simulink model "z8"  (R2023b)
settings: Solver=FixedStepAuto  StartTime=0.0  StopTime=10.0  FixedStep=0.01  RelTol=1e-3
values from neighbouring files (symbols this model uses):
  C = q_bar * S * C_C    [z8.m]
  D = q_bar * S * C_D    [z8.m]
  L = q_bar * S * C_L    [z8.m]
undefined symbols (not defined in the file or in its folder): Ix, Iy, Iz, l_AB, m_AB, n_AB
settings Model: Creator=asus  LastModifiedBy=asus

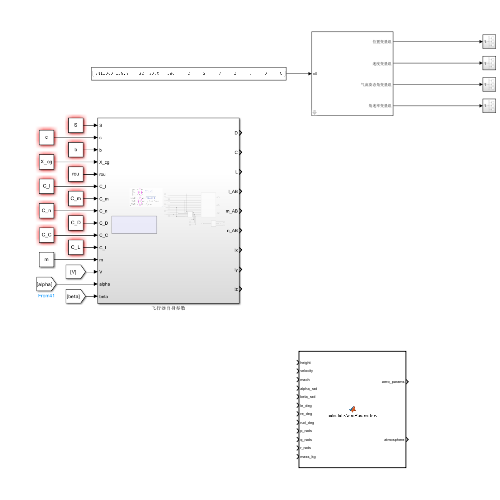
[thumbnail: Simulink's stored preview of the top-level diagram]
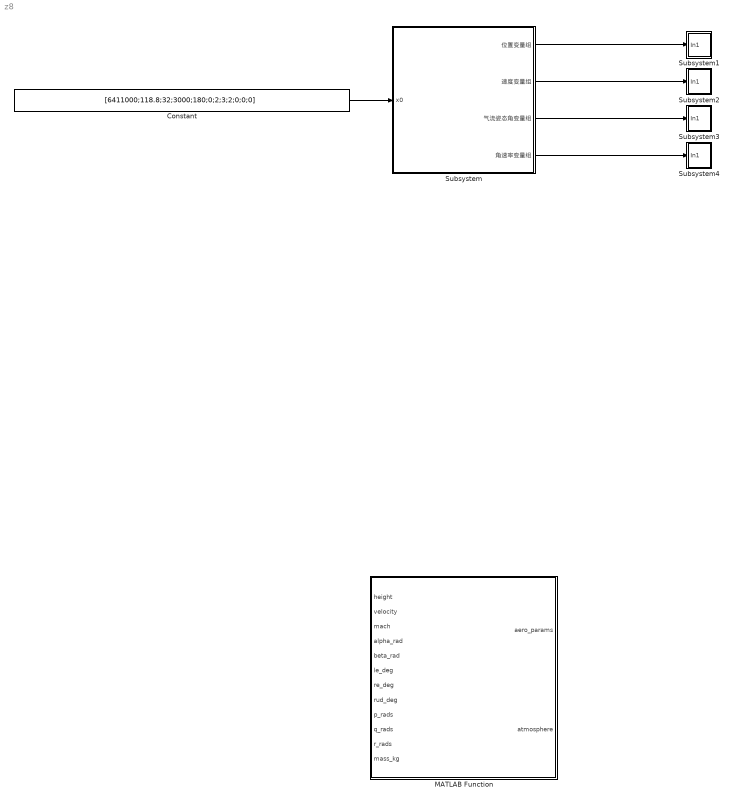
== system z8 ==
  Constant : Constant  Value=[6411000;118.8;32;3000;180;0;2;3;2;0;0;0]
  MATLAB Function : MATLAB Function  TreatAsAtomicUnit=on
  Subsystem : Subsystem  mask{m=136820, g=9.65, w_E=7.3*1e-5, S=334.73, c=24.384, b=18.288, rou=0, C_I=0, C_m=0, C_n=0, C_D=0, C_C=0, C_L=0}
      mask prompts: m "m质量"; g "g重力加速度"; w_E "w_E地球自转角速度"; S "S机翼面积"; c "c平均气动弦长"; b "b机翼展长"; C_I "C_l"
      mask DialogControl ParameterGroupVar Prompt: 参数
  Subsystem1 : Subsystem
  Subsystem2 : Subsystem
  Subsystem3 : Subsystem
  Subsystem4 : Subsystem
  wires:
  Constant/1 -> Subsystem/1(x0)
  Subsystem/2(速度变量组) -> Subsystem2/1(In1)
  Subsystem/4(角速率变量组) -> Subsystem4/1(In1)
  Subsystem/1(位置变量组) -> Subsystem1/1(In1)
  Subsystem/3(气流姿态角变量组) -> Subsystem3/1(In1)

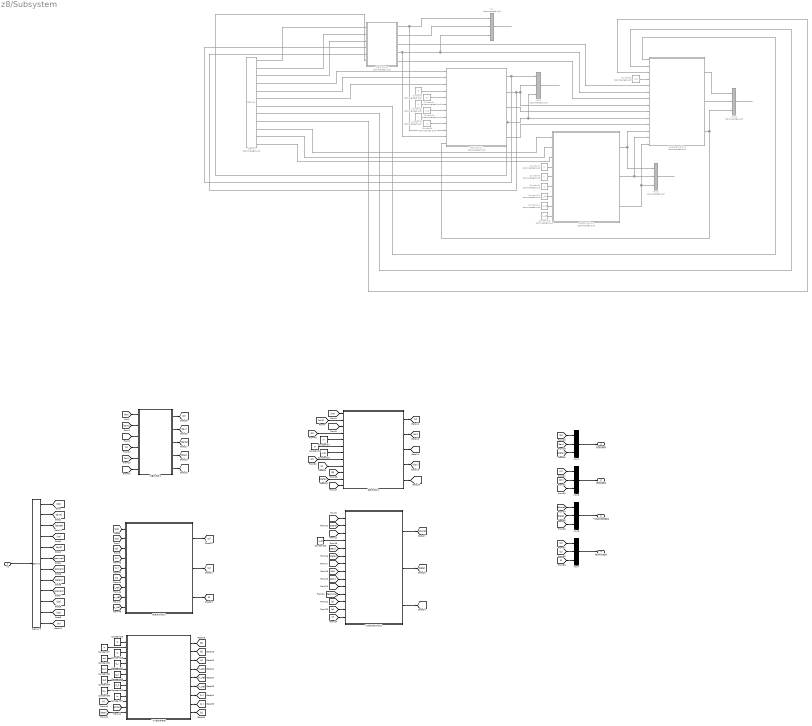
== system z8/Subsystem ==
  x0 : Inport
  Constant : Constant  Commented=on  Value=D
  Constant1 : Constant  Commented=on  Value=m
  Constant10 : Constant  Commented=on  Value=l_AB
  Constant11 : Constant  Commented=on  Value=m_AB
  Constant12 : Constant  Commented=on  Value=n_AB
  Constant14 : Constant  Value=m
  Constant18 : Constant  Value=g
  Constant19 : Constant  Value=w_E
  Constant2 : Constant  Commented=on  Value=g
  Constant22 : Constant  Value=w_E
  Constant26 : Constant  Value=S
  Constant27 : Constant  Value=c
  Constant28 : Constant  Value=b
  Constant3 : Constant  Commented=on  Value=w_E
  Constant30 : Constant  Value=rou
  Constant31 : Constant  Value=C_I
  Constant32 : Constant  Value=C_m
  Constant33 : Constant  Value=C_n
  Constant34 : Constant  Value=C_D
  Constant35 : Constant  Value=C_C
  Constant36 : Constant  Value=C_L
  Constant37 : Constant  Value=m
  Constant4 : Constant  Commented=on  Value=L
  Constant5 : Constant  Commented=on  Value=C
  Constant6 : Constant  Commented=on  Value=w_E
  Constant7 : Constant  Commented=on  Value=Ix
  Constant8 : Constant  Commented=on  Value=Iy
  Constant9 : Constant  Commented=on  Value=Iz
  Demux : Demux  Commented=on  Outputs=12
  Demux1 : Demux  Outputs=12
  Mux{,1..3} (4 alike) : Mux  Commented=on  Inputs=3
  Mux{4..7} (4 alike) : Mux  Inputs=3
  位置方程组1 : Subsystem
  位置方程组12 : Subsystem  Commented=on
  气流姿态角方程组1 : Subsystem
  气流姿态角方程组12 : Subsystem  Commented=on
  角速率方程组1 : Subsystem
  角速率方程组12 : Subsystem  Commented=on
  速度方程组1 : Subsystem
  速度方程组12 : Subsystem  Commented=on
  飞行器自身参数 : Subsystem
  位置变量组 : Outport
  速度变量组 : Outport  Port=2
  气流姿态角变量组 : Outport  Port=3
  角速率变量组 : Outport  Port=4
  wires:
  气流姿态角方程组12/2(beta) -> Mux2/2
  角速率方程组12/1(p) -> Mux3/1, 气流姿态角方程组12/12(p)
  Constant12/1 -> 角速率方程组12/9(n_AB)
  Demux/11 -> 角速率方程组12/2(q0)
  Constant2/1 -> 速度方程组12/6(g)
  位置方程组12/1(R) -> Mux/1, 速度方程组12/10(R)
  角速率方程组12/2(q) -> Mux3/2, 气流姿态角方程组12/13(q)
  Demux/5 -> 速度方程组12/2(chi0)
  Demux/1 -> 位置方程组12/1(R0)
  位置方程组12/4(delta) -> 气流姿态角方程组12/6(delta), Mux/3, 速度方程组12/11(delta)
  速度方程组12/1(V) -> 位置方程组12/4(V), Mux1/1
  Constant4/1 -> 速度方程组12/8(L)
  Mux2/1 -> ?
  角速率方程组12/3(r) -> Mux3/3, 气流姿态角方程组12/14(r)
  Constant8/1 -> 角速率方程组12/5(Iy)
  Demux/2 -> 位置方程组12/2(tau0)
  速度方程组12/2(chi) -> 位置方程组12/5(chi), Mux1/2, 气流姿态角方程组12/8(chi)
  气流姿态角方程组12/1(alpha) -> Mux2/1
  气流姿态角方程组12/3(sigma) -> Mux2/3, 速度方程组12/12(sigma)
  速度方程组12/4(gamma) -> 位置方程组12/6(gamma), Mux1/3, 气流姿态角方程组12/10(gamma)
  Mux3/1 -> ?
  位置方程组12/2(tau) -> Mux/2
  Constant7/1 -> 角速率方程组12/4(Ix)
  Demux/6 -> 速度方程组12/3(gamma0)
  Constant1/1 -> 速度方程组12/5(m)
  Demux/10 -> 角速率方程组12/1(p0)
  速度方程组12/5(dgamma) -> 气流姿态角方程组12/11(dgamma)
  Constant11/1 -> 角速率方程组12/8(m_AB)
  位置方程组12/3(dtau) -> 气流姿态角方程组12/5(dtau)
  Demux/4 -> 速度方程组12/1(V0)
  Mux1/1 -> ?
  Demux/12 -> 角速率方程组12/3(r0)
  位置方程组12/5(dddelta) -> 气流姿态角方程组12/7(ddelta)
  速度方程组12/3(dchi) -> 气流姿态角方程组12/9(dchi)
  Constant5/1 -> 速度方程组12/9(C)
  Constant6/1 -> 气流姿态角方程组12/4(w_E)
  Constant/1 -> 速度方程组12/4(D)
  Constant9/1 -> 角速率方程组12/6(Iz)
  Demux/8 -> 气流姿态角方程组12/2(beta0)
  Mux/1 -> ?
  Constant3/1 -> 速度方程组12/7(w_E)
  Constant10/1 -> 角速率方程组12/7(l_AB)
  Demux/9 -> 气流姿态角方程组12/3(sigma0)
  ? -> Demux/1
  Demux/3 -> 位置方程组12/3(delta0)
  Demux/7 -> 气流姿态角方程组12/1(alpha0)
  [C] -> 速度方程组1/8(L)
  Mux5/1 -> 速度变量组/1
  x0/1 -> Demux1/1
  Constant22/1 -> 气流姿态角方程组1/4(w_E)
  [Ix] -> 角速率方程组1/4(Ix)
  Mux7/1 -> 角速率变量组/1
  [L] -> 速度方程组1/9(C)
  Constant14/1 -> 速度方程组1/5(m)
  Constant19/1 -> 速度方程组1/7(w_E)
  Mux6/1 -> 气流姿态角变量组/1
  [D] -> 速度方程组1/4(D)
  Constant18/1 -> 速度方程组1/6(g)
  Demux1/1 -> [R0]
  Demux1/2 -> [tau0]
  Demux1/3 -> [delta0]
  Demux1/4 -> [V0]
  Demux1/5 -> [chi0]
  Demux1/6 -> [gamma0]
  Demux1/7 -> [alpha0]
  Demux1/8 -> [beta0]
  Demux1/9 -> [sigma0]
  Demux1/10 -> [p0]
  Demux1/11 -> [q0]
  Demux1/12 -> [r0]
  [R0] -> 位置方程组1/1(R0)
  [tau0] -> 位置方程组1/2(tau0)
  [delta0] -> 位置方程组1/3(delta0)
  [V0] -> 速度方程组1/1(V0)
  [chi0] -> 速度方程组1/2(chi0)
  [gamma0] -> 速度方程组1/3(gamma0)
  [p0] -> 角速率方程组1/1(p0)
  [q0] -> 角速率方程组1/2(q0)
  [r0] -> 角速率方程组1/3(r0)
  [alpha0] -> 气流姿态角方程组1/1(alpha0)
  [beta0] -> 气流姿态角方程组1/2(beta0)
  [sigma0] -> 气流姿态角方程组1/3(sigma0)
  速度方程组1/1(V) -> [V]
  速度方程组1/2(chi) -> [chi]
  速度方程组1/3(gamma) -> [gamma]
  [V] -> 位置方程组1/4(V)
  [chi] -> 位置方程组1/5(chi)
  [gamma] -> 位置方程组1/6(gamma)
  位置方程组1/4(dtau) -> [dtau]
  位置方程组1/5(dddelta) -> [ddelta]
  位置方程组1/3(delta) -> [delta]
  位置方程组1/1(R) -> [R]
  [dtau] -> 气流姿态角方程组1/5(dtau)
  [delta] -> 气流姿态角方程组1/6(delta)
  [ddelta] -> 气流姿态角方程组1/7(ddelta)
  [chi] -> 气流姿态角方程组1/8(chi)
  [dchi] -> 气流姿态角方程组1/9(dchi)
  速度方程组1/4(dchi) -> [dchi]
  速度方程组1/5(dgamma) -> [dgamma]
  [gamma] -> 气流姿态角方程组1/10(gamma)
  [dgamma] -> 气流姿态角方程组1/11(dgamma)
  角速率方程组1/1(p) -> [p]
  角速率方程组1/2(q) -> [q]
  角速率方程组1/3(r) -> [r]
  [p] -> 气流姿态角方程组1/12(p)
  [q] -> 气流姿态角方程组1/13(q)
  [r] -> 气流姿态角方程组1/14(r)
  [R] -> 速度方程组1/10(R)
  [delta] -> 速度方程组1/11(delta)
  [sigma] -> 速度方程组1/12(sigma)
  气流姿态角方程组1/3(sigma) -> [sigma]
  位置方程组1/2(tau) -> [tau]
  气流姿态角方程组1/2(beta) -> [beta]
  气流姿态角方程组1/1(alpha) -> [alpha]
  Mux4/1 -> 位置变量组/1
  [R] -> Mux4/1
  [tau] -> Mux4/2
  [delta] -> Mux4/3
  [V] -> Mux5/1
  [chi] -> Mux5/2
  [gamma] -> Mux5/3
  [alpha] -> Mux6/1
  [beta] -> Mux6/2
  [sigma] -> Mux6/3
  [p] -> Mux7/1
  [q] -> Mux7/2
  [r] -> Mux7/3
  Constant26/1 -> 飞行器自身参数/1(S)
  Constant27/1 -> 飞行器自身参数/2(c)
  Constant28/1 -> 飞行器自身参数/3(b)
  Constant30/1 -> 飞行器自身参数/4(rou)
  Constant31/1 -> 飞行器自身参数/5(C_l)
  Constant32/1 -> 飞行器自身参数/6(C_m)
  Constant33/1 -> 飞行器自身参数/7(C_n)
  Constant34/1 -> 飞行器自身参数/8(C_D)
  Constant35/1 -> 飞行器自身参数/9(C_C)
  Constant36/1 -> 飞行器自身参数/10(C_L)
  Constant37/1 -> 飞行器自身参数/11(m)
  [V] -> 飞行器自身参数/12(V)
  [alpha] -> 飞行器自身参数/13(alpha)
  [beta] -> 飞行器自身参数/14(beta)
  飞行器自身参数/1(D) -> [D]
  飞行器自身参数/2(C) -> [C]
  飞行器自身参数/3(L) -> [L]
  飞行器自身参数/4(l_AB) -> [l_AB]
  飞行器自身参数/5(m_AB) -> [m_AB]
  飞行器自身参数/6(n_AB) -> [n_AB]
  飞行器自身参数/7(Ix) -> [Ix]
  飞行器自身参数/8(Iy) -> [Iy]
  飞行器自身参数/9(Iz) -> [Iz]
  [Iy] -> 角速率方程组1/5(Iy)
  [Iz] -> 角速率方程组1/6(Iz)
  [l_AB] -> 角速率方程组1/7(l_AB)
  [m_AB] -> 角速率方程组1/8(m_AB)
  [n_AB] -> 角速率方程组1/9(n_AB)

== system z8/Subsystem1 ==
  In1 : Inport
  Demux : Demux  Outputs=3
  Scope4 : Scope
  Scope5 : Scope
  Scope6 : Scope
  wires:
  In1/1 -> Demux/1
  Demux/1 -> Scope4/1
  Demux/2 -> Scope5/1
  Demux/3 -> Scope6/1

== system z8/Subsystem2 ==
  In1 : Inport
  Demux : Demux  Outputs=3
  Scope4 : Scope
  Scope5 : Scope
  Scope6 : Scope
  wires:
  Demux/3 -> Scope6/1
  Demux/2 -> Scope5/1
  Demux/1 -> Scope4/1
  In1/1 -> Demux/1

== system z8/Subsystem3 ==
  In1 : Inport
  Demux : Demux  Outputs=3
  Scope4 : Scope
  Scope5 : Scope
  Scope6 : Scope
  wires:
  In1/1 -> Demux/1
  Demux/1 -> Scope4/1
  Demux/2 -> Scope5/1
  Demux/3 -> Scope6/1

== system z8/Subsystem4 ==
  In1 : Inport
  Demux : Demux  Outputs=3
  Scope4 : Scope
  Scope5 : Scope
  Scope6 : Scope
  wires:
  Demux/3 -> Scope6/1
  Demux/2 -> Scope5/1
  Demux/1 -> Scope4/1
  In1/1 -> Demux/1

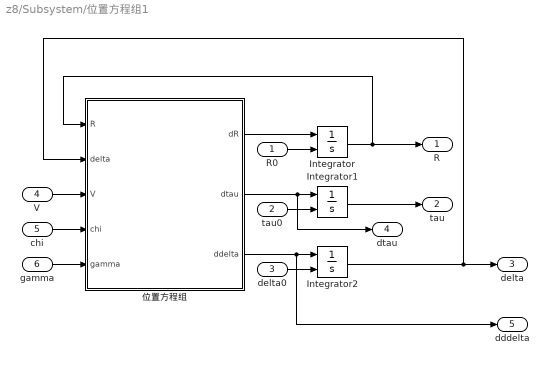
== system z8/Subsystem/位置方程组1 ==
  R0 : Inport
  tau0 : Inport  Port=2
  delta0 : Inport  Port=3
  V : Inport  Port=4
  chi : Inport  Port=5
  gamma : Inport  Port=6
  Integrator : Integrator  InitialConditionSource=external
  Integrator1 : Integrator  InitialConditionSource=external
  Integrator2 : Integrator  InitialConditionSource=external
  位置方程组 : MATLAB Function  TreatAsAtomicUnit=on
  R : Outport
  tau : Outport  Port=2
  delta : Outport  Port=3
  dtau : Outport  Port=4
  dddelta : Outport  Port=5
  wires:
  Integrator2/1 -> delta/1, 位置方程组/2(delta)
  delta0/1 -> Integrator2/2
  Integrator/1 -> R/1, 位置方程组/1(R)
  chi/1 -> 位置方程组/4(chi)
  Integrator1/1 -> tau/1
  V/1 -> 位置方程组/3(V)
  位置方程组/2(dtau) -> dtau/1, Integrator1/1
  R0/1 -> Integrator/2
  位置方程组/3(ddelta) -> dddelta/1, Integrator2/1
  位置方程组/1(dR) -> Integrator/1
  tau0/1 -> Integrator1/2
  gamma/1 -> 位置方程组/5(gamma)

== system z8/Subsystem/位置方程组12 ==
  R0 : Inport
  tau0 : Inport  Port=2
  delta0 : Inport  Port=3
  V : Inport  Port=4
  chi : Inport  Port=5
  gamma : Inport  Port=6
  Integrator : Integrator  InitialConditionSource=external
  Integrator1 : Integrator  InitialConditionSource=external
  Integrator2 : Integrator  InitialConditionSource=external
  位置方程组 : MATLAB Function  TreatAsAtomicUnit=on
  R : Outport
  tau : Outport  Port=2
  dtau : Outport  Port=3
  delta : Outport  Port=4
  dddelta : Outport  Port=5
  wires:
  Integrator2/1 -> delta/1, 位置方程组/2(delta)
  delta0/1 -> Integrator2/2
  Integrator/1 -> R/1, 位置方程组/1(R)
  chi/1 -> 位置方程组/4(chi)
  Integrator1/1 -> tau/1
  V/1 -> 位置方程组/3(V)
  位置方程组/2(dtau) -> dtau/1, Integrator1/1
  R0/1 -> Integrator/2
  位置方程组/3(ddelta) -> dddelta/1, Integrator2/1
  位置方程组/1(dR) -> Integrator/1
  tau0/1 -> Integrator1/2
  gamma/1 -> 位置方程组/5(gamma)

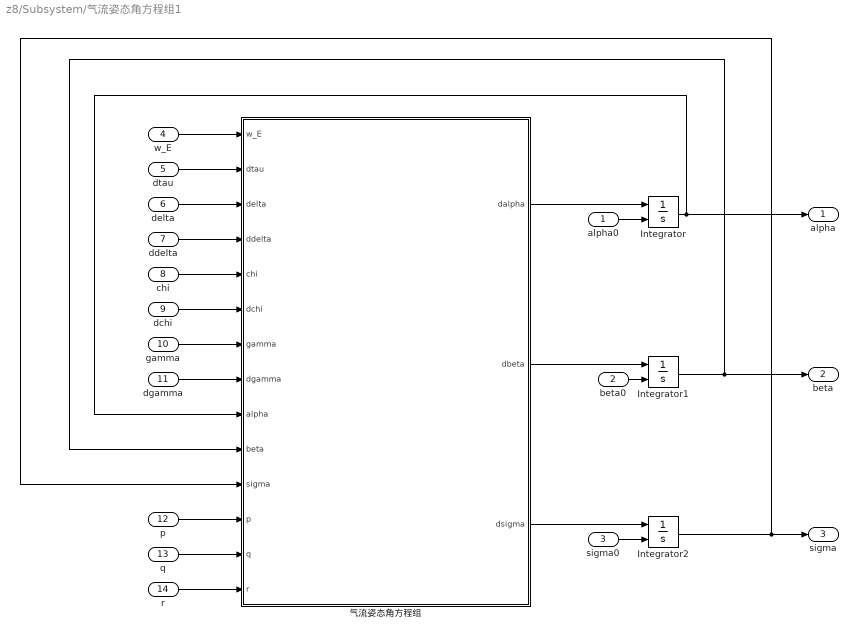
== system z8/Subsystem/气流姿态角方程组1 ==
  alpha0 : Inport
  beta0 : Inport  Port=2
  sigma0 : Inport  Port=3
  w_E : Inport  Port=4
  dtau : Inport  Port=5
  delta : Inport  Port=6
  ddelta : Inport  Port=7
  chi : Inport  Port=8
  dchi : Inport  Port=9
  gamma : Inport  Port=10
  dgamma : Inport  Port=11
  p : Inport  Port=12
  q : Inport  Port=13
  r : Inport  Port=14
  Integrator : Integrator  InitialConditionSource=external
  Integrator1 : Integrator  InitialConditionSource=external
  Integrator2 : Integrator  InitialConditionSource=external
  气流姿态角方程组 : Subsystem
  alpha : Outport
  beta : Outport  Port=2
  sigma : Outport  Port=3
  wires:
  气流姿态角方程组/3(dsigma) -> Integrator2/1
  Integrator/1 -> alpha/1, 气流姿态角方程组/9(alpha)
  r/1 -> 气流姿态角方程组/14(r)
  q/1 -> 气流姿态角方程组/13(q)
  ddelta/1 -> 气流姿态角方程组/4(ddelta)
  gamma/1 -> 气流姿态角方程组/7(gamma)
  dchi/1 -> 气流姿态角方程组/6(dchi)
  Integrator1/1 -> beta/1, 气流姿态角方程组/10(beta)
  sigma0/1 -> Integrator2/2
  Integrator2/1 -> sigma/1, 气流姿态角方程组/11(sigma)
  dgamma/1 -> 气流姿态角方程组/8(dgamma)
  chi/1 -> 气流姿态角方程组/5(chi)
  p/1 -> 气流姿态角方程组/12(p)
  dtau/1 -> 气流姿态角方程组/2(dtau)
  delta/1 -> 气流姿态角方程组/3(delta)
  气流姿态角方程组/2(dbeta) -> Integrator1/1
  w_E/1 -> 气流姿态角方程组/1(w_E)
  alpha0/1 -> Integrator/2
  气流姿态角方程组/1(dalpha) -> Integrator/1
  beta0/1 -> Integrator1/2

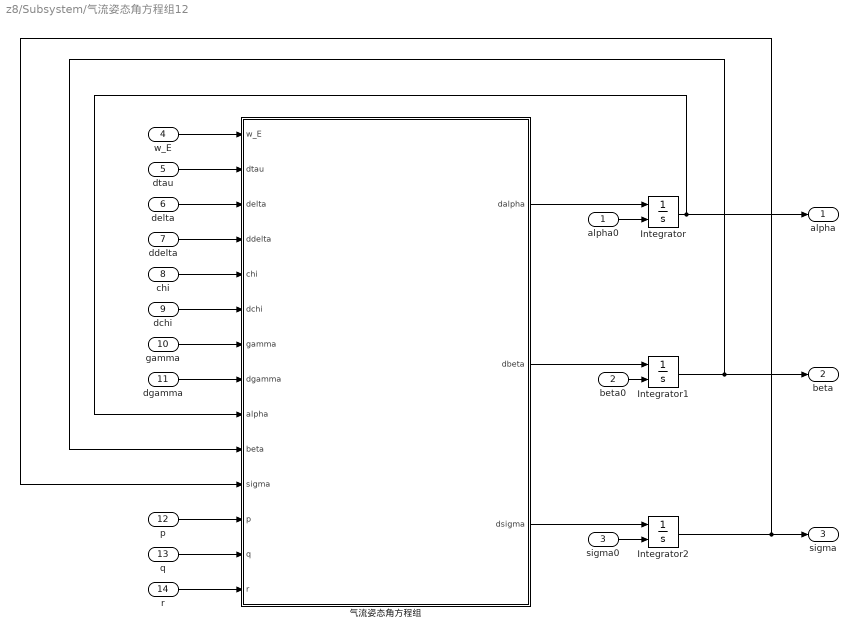
== system z8/Subsystem/气流姿态角方程组12 ==
  alpha0 : Inport
  beta0 : Inport  Port=2
  sigma0 : Inport  Port=3
  w_E : Inport  Port=4
  dtau : Inport  Port=5
  delta : Inport  Port=6
  ddelta : Inport  Port=7
  chi : Inport  Port=8
  dchi : Inport  Port=9
  gamma : Inport  Port=10
  dgamma : Inport  Port=11
  p : Inport  Port=12
  q : Inport  Port=13
  r : Inport  Port=14
  Integrator : Integrator  InitialConditionSource=external
  Integrator1 : Integrator  InitialConditionSource=external
  Integrator2 : Integrator  InitialConditionSource=external
  气流姿态角方程组 : Subsystem
  alpha : Outport
  beta : Outport  Port=2
  sigma : Outport  Port=3
  wires:
  气流姿态角方程组/3(dsigma) -> Integrator2/1
  Integrator/1 -> alpha/1, 气流姿态角方程组/9(alpha)
  r/1 -> 气流姿态角方程组/14(r)
  q/1 -> 气流姿态角方程组/13(q)
  ddelta/1 -> 气流姿态角方程组/4(ddelta)
  gamma/1 -> 气流姿态角方程组/7(gamma)
  dchi/1 -> 气流姿态角方程组/6(dchi)
  Integrator1/1 -> beta/1, 气流姿态角方程组/10(beta)
  sigma0/1 -> Integrator2/2
  Integrator2/1 -> sigma/1, 气流姿态角方程组/11(sigma)
  dgamma/1 -> 气流姿态角方程组/8(dgamma)
  chi/1 -> 气流姿态角方程组/5(chi)
  p/1 -> 气流姿态角方程组/12(p)
  dtau/1 -> 气流姿态角方程组/2(dtau)
  delta/1 -> 气流姿态角方程组/3(delta)
  气流姿态角方程组/2(dbeta) -> Integrator1/1
  w_E/1 -> 气流姿态角方程组/1(w_E)
  alpha0/1 -> Integrator/2
  气流姿态角方程组/1(dalpha) -> Integrator/1
  beta0/1 -> Integrator1/2

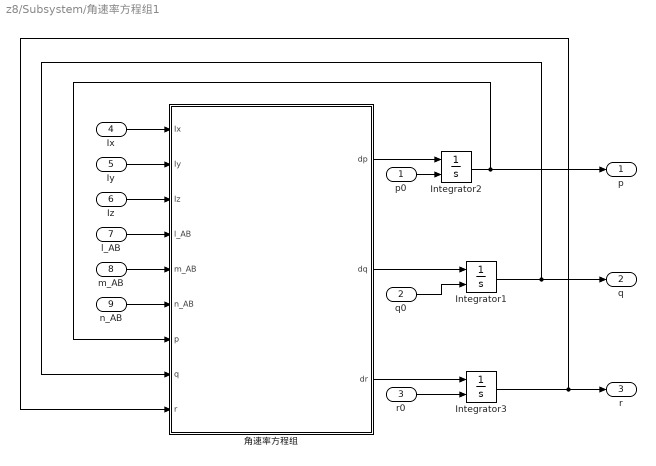
== system z8/Subsystem/角速率方程组1 ==
  p0 : Inport
  q0 : Inport  Port=2
  r0 : Inport  Port=3
  Ix : Inport  Port=4
  Iy : Inport  Port=5
  Iz : Inport  Port=6
  l_AB : Inport  Port=7
  m_AB : Inport  Port=8
  n_AB : Inport  Port=9
  Integrator1 : Integrator  InitialConditionSource=external
  Integrator2 : Integrator  InitialConditionSource=external
  Integrator3 : Integrator  InitialConditionSource=external
  角速率方程组 : MATLAB Function  TreatAsAtomicUnit=on
  p : Outport
  q : Outport  Port=2
  r : Outport  Port=3
  wires:
  Iy/1 -> 角速率方程组/2(Iy)
  Ix/1 -> 角速率方程组/1(Ix)
  n_AB/1 -> 角速率方程组/6(n_AB)
  q0/1 -> Integrator1/2
  Integrator3/1 -> r/1, 角速率方程组/9(r)
  Integrator1/1 -> q/1, 角速率方程组/8(q)
  角速率方程组/3(dr) -> Integrator3/1
  r0/1 -> Integrator3/2
  Integrator2/1 -> p/1, 角速率方程组/7(p)
  角速率方程组/2(dq) -> Integrator1/1
  p0/1 -> Integrator2/2
  角速率方程组/1(dp) -> Integrator2/1
  Iz/1 -> 角速率方程组/3(Iz)
  m_AB/1 -> 角速率方程组/5(m_AB)
  l_AB/1 -> 角速率方程组/4(l_AB)

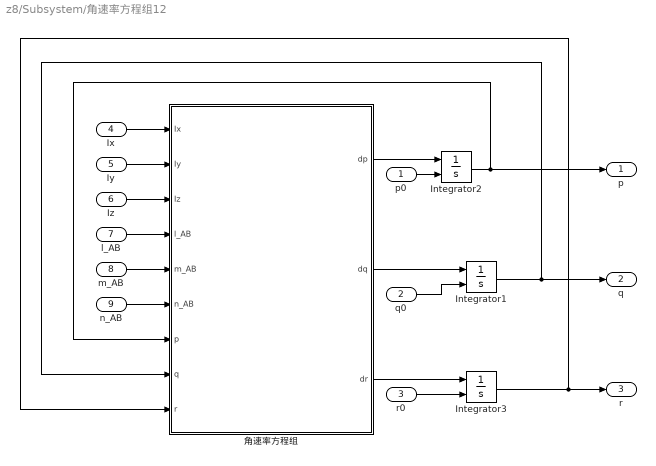
== system z8/Subsystem/角速率方程组12 ==
  p0 : Inport
  q0 : Inport  Port=2
  r0 : Inport  Port=3
  Ix : Inport  Port=4
  Iy : Inport  Port=5
  Iz : Inport  Port=6
  l_AB : Inport  Port=7
  m_AB : Inport  Port=8
  n_AB : Inport  Port=9
  Integrator1 : Integrator  InitialConditionSource=external
  Integrator2 : Integrator  InitialConditionSource=external
  Integrator3 : Integrator  InitialConditionSource=external
  角速率方程组 : MATLAB Function  TreatAsAtomicUnit=on
  p : Outport
  q : Outport  Port=2
  r : Outport  Port=3
  wires:
  Iy/1 -> 角速率方程组/2(Iy)
  Ix/1 -> 角速率方程组/1(Ix)
  n_AB/1 -> 角速率方程组/6(n_AB)
  q0/1 -> Integrator1/2
  Integrator3/1 -> r/1, 角速率方程组/9(r)
  Integrator1/1 -> q/1, 角速率方程组/8(q)
  角速率方程组/3(dr) -> Integrator3/1
  r0/1 -> Integrator3/2
  Integrator2/1 -> p/1, 角速率方程组/7(p)
  角速率方程组/2(dq) -> Integrator1/1
  p0/1 -> Integrator2/2
  角速率方程组/1(dp) -> Integrator2/1
  Iz/1 -> 角速率方程组/3(Iz)
  m_AB/1 -> 角速率方程组/5(m_AB)
  l_AB/1 -> 角速率方程组/4(l_AB)

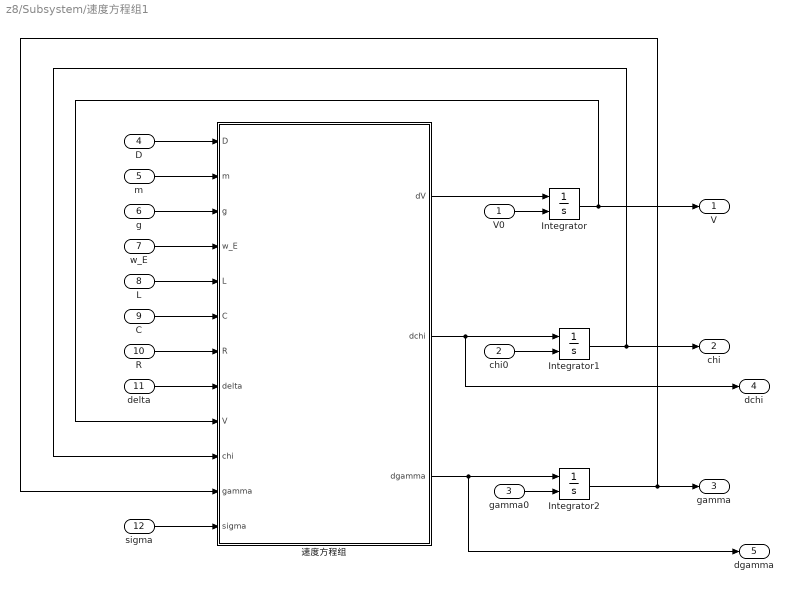
== system z8/Subsystem/速度方程组1 ==
  V0 : Inport
  chi0 : Inport  Port=2
  gamma0 : Inport  Port=3
  D : Inport  Port=4
  m : Inport  Port=5
  g : Inport  Port=6
  w_E : Inport  Port=7
  L : Inport  Port=8
  C : Inport  Port=9
  R : Inport  Port=10
  delta : Inport  Port=11
  sigma : Inport  Port=12
  Integrator : Integrator  InitialConditionSource=external
  Integrator1 : Integrator  InitialConditionSource=external
  Integrator2 : Integrator  InitialConditionSource=external
  速度方程组 : MATLAB Function  TreatAsAtomicUnit=on
  V : Outport
  chi : Outport  Port=2
  gamma : Outport  Port=3
  dchi : Outport  Port=4
  dgamma : Outport  Port=5
  wires:
  Integrator2/1 -> gamma/1, 速度方程组/11(gamma)
  R/1 -> 速度方程组/7(R)
  速度方程组/2(dchi) -> dchi/1, Integrator1/1
  Integrator/1 -> V/1, 速度方程组/9(V)
  速度方程组/3(dgamma) -> Integrator2/1, dgamma/1
  L/1 -> 速度方程组/5(L)
  速度方程组/1(dV) -> Integrator/1
  m/1 -> 速度方程组/2(m)
  g/1 -> 速度方程组/3(g)
  sigma/1 -> 速度方程组/12(sigma)
  delta/1 -> 速度方程组/8(delta)
  chi0/1 -> Integrator1/2
  C/1 -> 速度方程组/6(C)
  V0/1 -> Integrator/2
  gamma0/1 -> Integrator2/2
  D/1 -> 速度方程组/1(D)
  Integrator1/1 -> chi/1, 速度方程组/10(chi)
  w_E/1 -> 速度方程组/4(w_E)

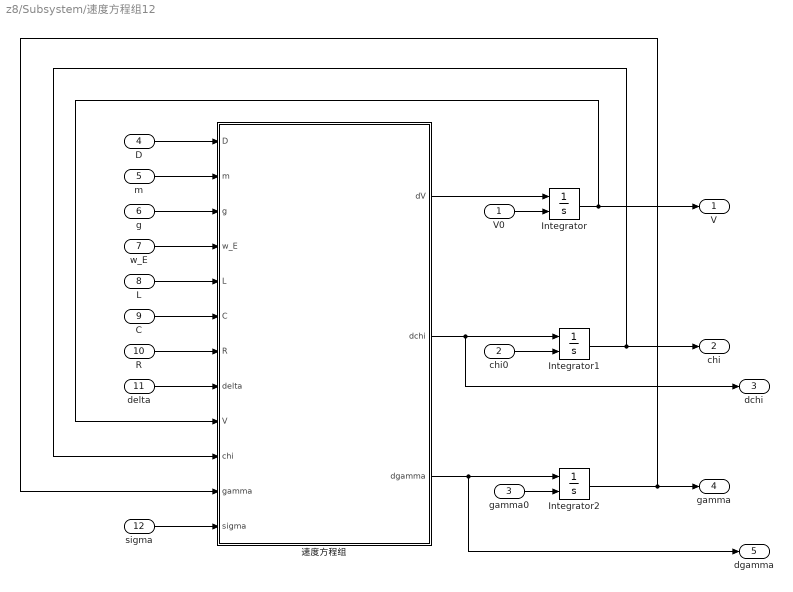
== system z8/Subsystem/速度方程组12 ==
  V0 : Inport
  chi0 : Inport  Port=2
  gamma0 : Inport  Port=3
  D : Inport  Port=4
  m : Inport  Port=5
  g : Inport  Port=6
  w_E : Inport  Port=7
  L : Inport  Port=8
  C : Inport  Port=9
  R : Inport  Port=10
  delta : Inport  Port=11
  sigma : Inport  Port=12
  Integrator : Integrator  InitialConditionSource=external
  Integrator1 : Integrator  InitialConditionSource=external
  Integrator2 : Integrator  InitialConditionSource=external
  速度方程组 : MATLAB Function  TreatAsAtomicUnit=on
  V : Outport
  chi : Outport  Port=2
  dchi : Outport  Port=3
  gamma : Outport  Port=4
  dgamma : Outport  Port=5
  wires:
  Integrator2/1 -> gamma/1, 速度方程组/11(gamma)
  R/1 -> 速度方程组/7(R)
  速度方程组/2(dchi) -> dchi/1, Integrator1/1
  Integrator/1 -> V/1, 速度方程组/9(V)
  速度方程组/3(dgamma) -> Integrator2/1, dgamma/1
  L/1 -> 速度方程组/5(L)
  速度方程组/1(dV) -> Integrator/1
  m/1 -> 速度方程组/2(m)
  g/1 -> 速度方程组/3(g)
  sigma/1 -> 速度方程组/12(sigma)
  delta/1 -> 速度方程组/8(delta)
  chi0/1 -> Integrator1/2
  C/1 -> 速度方程组/6(C)
  V0/1 -> Integrator/2
  gamma0/1 -> Integrator2/2
  D/1 -> 速度方程组/1(D)
  Integrator1/1 -> chi/1, 速度方程组/10(chi)
  w_E/1 -> 速度方程组/4(w_E)

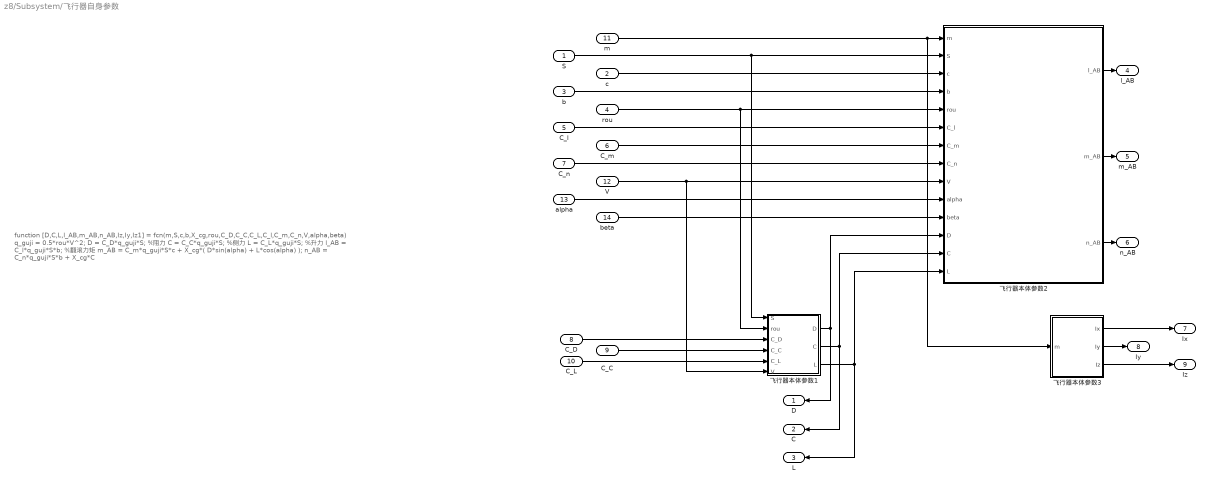
== system z8/Subsystem/飞行器自身参数 ==
  note: function [D,C,L,l_AB,m_AB,n_AB,Iz,Iy,Iz1] = fcn(m,S,c,b,X_cg,rou,C_D,C_C,C_L,C_l,C_m,C_n,V,alpha,beta)
      |
      | q_guji = 0.5*rou*V^2;
      |
      | D = C_D*q_guji*S;    %阻力
      | C = C_C*q_guji*S;    %侧力
      | L = C_L*q_guji*S;    %升力
      |
      | l_AB = C_l*q_guji*S*b;  %翻滚力矩
      | m_AB = C_m*q_guji*S*c + X_cg*( D*sin(alpha) + L*cos(alpha) );
      | n_AB = C_n*q_guji*S*b + X_cg*C
  S : Inport
  c : Inport  Port=2
  b : Inport  Port=3
  rou : Inport  Port=4
  C_l : Inport  Port=5
  C_m : Inport  Port=6
  C_n : Inport  Port=7
  C_D : Inport  Port=8
  C_C : Inport  Port=9
  C_L : Inport  Port=10
  m : Inport  Port=11
  V : Inport  Port=12
  alpha : Inport  Port=13
  beta : Inport  Port=14
  飞行器本体参数1 : MATLAB Function  TreatAsAtomicUnit=on
  飞行器本体参数2 : MATLAB Function  TreatAsAtomicUnit=on
  飞行器本体参数3 : MATLAB Function  TreatAsAtomicUnit=on
  D : Outport
  C : Outport  Port=2
  L : Outport  Port=3
  l_AB : Outport  Port=4
  m_AB : Outport  Port=5
  n_AB : Outport  Port=6
  Ix : Outport  Port=7
  Iy : Outport  Port=8
  Iz : Outport  Port=9
  wires:
  C_C/1 -> 飞行器本体参数1/4(C_C)
  飞行器本体参数1/3(L) -> L/1, 飞行器本体参数2/14(L)
  飞行器本体参数1/1(D) -> D/1, 飞行器本体参数2/12(D)
  C_D/1 -> 飞行器本体参数1/3(C_D)
  飞行器本体参数3/3(Iz) -> Iz/1
  飞行器本体参数1/2(C) -> C/1, 飞行器本体参数2/13(C)
  S/1 -> 飞行器本体参数2/2(S), 飞行器本体参数1/1(S)
  b/1 -> 飞行器本体参数2/4(b)
  V/1 -> 飞行器本体参数1/6(V), 飞行器本体参数2/9(V)
  飞行器本体参数2/2(m_AB) -> m_AB/1
  C_L/1 -> 飞行器本体参数1/5(C_L)
  c/1 -> 飞行器本体参数2/3(c)
  C_m/1 -> 飞行器本体参数2/7(C_m)
  m/1 -> 飞行器本体参数3/1(m), 飞行器本体参数2/1(m)
  C_l/1 -> 飞行器本体参数2/6(C_l)
  C_n/1 -> 飞行器本体参数2/8(C_n)
  alpha/1 -> 飞行器本体参数2/10(alpha)
  beta/1 -> 飞行器本体参数2/11(beta)
  飞行器本体参数2/1(l_AB) -> l_AB/1
  rou/1 -> 飞行器本体参数2/5(rou), 飞行器本体参数1/2(rou)
  飞行器本体参数2/3(n_AB) -> n_AB/1
  飞行器本体参数3/1(Ix) -> Ix/1
  飞行器本体参数3/2(Iy) -> Iy/1

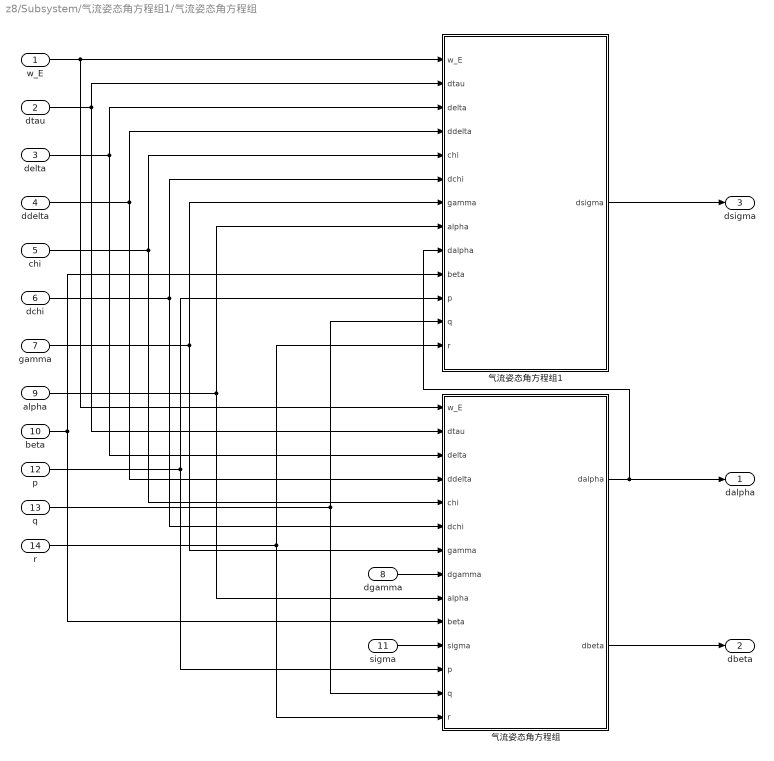
== system z8/Subsystem/气流姿态角方程组1/气流姿态角方程组 ==
  w_E : Inport
  dtau : Inport  Port=2
  delta : Inport  Port=3
  ddelta : Inport  Port=4
  chi : Inport  Port=5
  dchi : Inport  Port=6
  gamma : Inport  Port=7
  dgamma : Inport  Port=8
  alpha : Inport  Port=9
  beta : Inport  Port=10
  sigma : Inport  Port=11
  p : Inport  Port=12
  q : Inport  Port=13
  r : Inport  Port=14
  气流姿态角方程组 : MATLAB Function  TreatAsAtomicUnit=on
  气流姿态角方程组1 : MATLAB Function  TreatAsAtomicUnit=on
  dalpha : Outport
  dbeta : Outport  Port=2
  dsigma : Outport  Port=3
  wires:
  q/1 -> 气流姿态角方程组/13(q), 气流姿态角方程组1/12(q)
  dtau/1 -> 气流姿态角方程组/2(dtau), 气流姿态角方程组1/2(dtau)
  gamma/1 -> 气流姿态角方程组/7(gamma), 气流姿态角方程组1/7(gamma)
  chi/1 -> 气流姿态角方程组/5(chi), 气流姿态角方程组1/5(chi)
  alpha/1 -> 气流姿态角方程组/9(alpha), 气流姿态角方程组1/8(alpha)
  r/1 -> 气流姿态角方程组/14(r), 气流姿态角方程组1/13(r)
  dchi/1 -> 气流姿态角方程组/6(dchi), 气流姿态角方程组1/6(dchi)
  气流姿态角方程组/1(dalpha) -> dalpha/1, 气流姿态角方程组1/9(dalpha)
  w_E/1 -> 气流姿态角方程组/1(w_E), 气流姿态角方程组1/1(w_E)
  p/1 -> 气流姿态角方程组/12(p), 气流姿态角方程组1/11(p)
  气流姿态角方程组/2(dbeta) -> dbeta/1
  气流姿态角方程组1/1(dsigma) -> dsigma/1
  ddelta/1 -> 气流姿态角方程组/4(ddelta), 气流姿态角方程组1/4(ddelta)
  beta/1 -> 气流姿态角方程组/10(beta), 气流姿态角方程组1/10(beta)
  delta/1 -> 气流姿态角方程组/3(delta), 气流姿态角方程组1/3(delta)
  dgamma/1 -> 气流姿态角方程组/8(dgamma)
  sigma/1 -> 气流姿态角方程组/11(sigma)

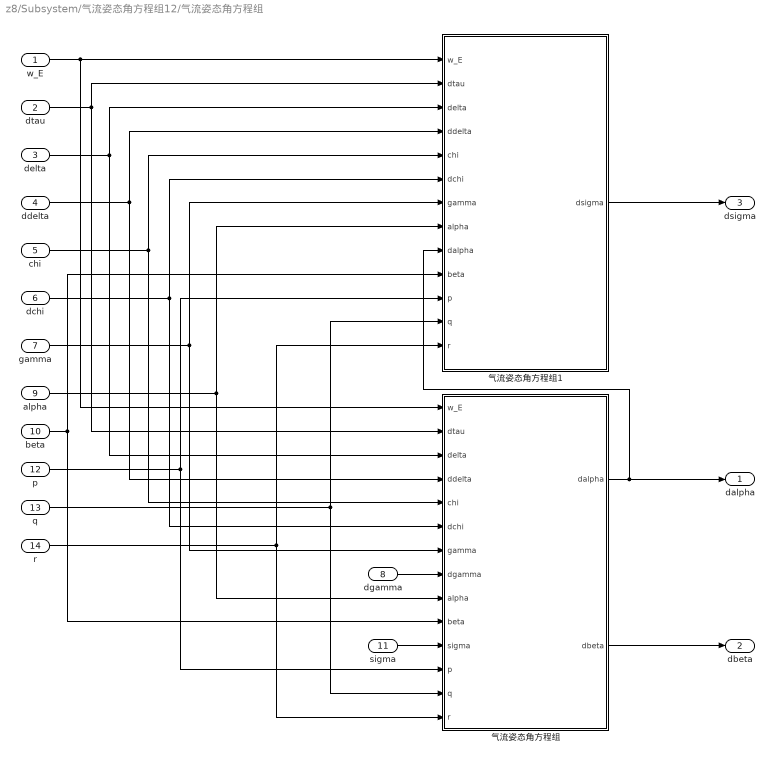
== system z8/Subsystem/气流姿态角方程组12/气流姿态角方程组 ==
  w_E : Inport
  dtau : Inport  Port=2
  delta : Inport  Port=3
  ddelta : Inport  Port=4
  chi : Inport  Port=5
  dchi : Inport  Port=6
  gamma : Inport  Port=7
  dgamma : Inport  Port=8
  alpha : Inport  Port=9
  beta : Inport  Port=10
  sigma : Inport  Port=11
  p : Inport  Port=12
  q : Inport  Port=13
  r : Inport  Port=14
  气流姿态角方程组 : MATLAB Function  TreatAsAtomicUnit=on
  气流姿态角方程组1 : MATLAB Function  TreatAsAtomicUnit=on
  dalpha : Outport
  dbeta : Outport  Port=2
  dsigma : Outport  Port=3
  wires:
  q/1 -> 气流姿态角方程组/13(q), 气流姿态角方程组1/12(q)
  dtau/1 -> 气流姿态角方程组/2(dtau), 气流姿态角方程组1/2(dtau)
  gamma/1 -> 气流姿态角方程组/7(gamma), 气流姿态角方程组1/7(gamma)
  chi/1 -> 气流姿态角方程组/5(chi), 气流姿态角方程组1/5(chi)
  alpha/1 -> 气流姿态角方程组/9(alpha), 气流姿态角方程组1/8(alpha)
  r/1 -> 气流姿态角方程组/14(r), 气流姿态角方程组1/13(r)
  dchi/1 -> 气流姿态角方程组/6(dchi), 气流姿态角方程组1/6(dchi)
  气流姿态角方程组/1(dalpha) -> dalpha/1, 气流姿态角方程组1/9(dalpha)
  w_E/1 -> 气流姿态角方程组/1(w_E), 气流姿态角方程组1/1(w_E)
  p/1 -> 气流姿态角方程组/12(p), 气流姿态角方程组1/11(p)
  气流姿态角方程组/2(dbeta) -> dbeta/1
  气流姿态角方程组1/1(dsigma) -> dsigma/1
  ddelta/1 -> 气流姿态角方程组/4(ddelta), 气流姿态角方程组1/4(ddelta)
  beta/1 -> 气流姿态角方程组/10(beta), 气流姿态角方程组1/10(beta)
  delta/1 -> 气流姿态角方程组/3(delta), 气流姿态角方程组1/3(delta)
  dgamma/1 -> 气流姿态角方程组/8(dgamma)
  sigma/1 -> 气流姿态角方程组/11(sigma)

== matlab function z8/Subsystem/角速率方程组12/角速率方程组 ==
  data: Ix input; Iy input; Iz input; l_AB input; dp output; m_AB input; dq output; dr output; n_AB input; p input; q input; r input
function [dp,dq,dr] = fcn(Ix,Iy,Iz,l_AB,m_AB,n_AB,p,q,r)

dp = ( Iy-Iz )*q*r/Ix + l_AB/Ix;
dq = ( Iz-Ix )*p*r/Iy + m_AB/Iy;
dr = ( Iz-Ix )*p*q/Iz + n_AB/Iz;

== matlab function z8/Subsystem/位置方程组1/位置方程组 ==
  data: R input; delta input; V input; chi input; dR output; gamma input; dtau output; ddelta output
function [dR,dtau,ddelta] = fcn(R,delta,V,chi,gamma)

dR = V*sin(gamma);
dtau = V*cos(gamma) * sin(chi) / ( R*cos(delta) );
ddelta = V*cos(gamma) * cos(chi) / R;

== matlab function z8/Subsystem/气流姿态角方程组1/气流姿态角方程组/气流姿态角方程组 ==
  data: w_E input; dtau input; delta input; ddelta input; chi input; dchi input; gamma input; dgamma input; alpha input; beta input; dalpha output; sigma input; dbeta output; p input; q input; r input
function [dalpha,dbeta] = fcn(w_E,dtau,delta,ddelta,chi,dchi,gamma,dgamma,alpha,beta,sigma,p,q,r)

dalpha = q - ( p*cos(alpha) + r*sin(alpha) )*tan(beta) + ...
        sin(sigma) / cos(beta) *( dchi*cos(gamma) - ddelta*sin(chi)*sin(gamma) + ( dtau + w_E )*( cos(delta)*cos(chi)*sin(gamma) - sin(delta)*cos(gamma) ) ) - ...
        cos(sigma) / cos(beta) *( dgamma - ddelta*cos(chi) - ( dtau + w_E )*cos(delta)*sin(chi) );
dbeta = p*sin(alpha) - r*cos(alpha) + sin(sigma)*( dgamma - ddelta*cos(chi) - ( dtau + w_E )*cos(delta)*sin(chi) ) + ...
        cos(sigma)*( dchi*cos(gamma) - ddelta*sin(chi)*sin(gamma) + ( dtau + w_E )*( cos(delta)*cos(chi)*sin(gamma) - sin(delta)*cos(gamma) ) );

== matlab function z8/Subsystem/气流姿态角方程组1/气流姿态角方程组/气流姿态角方程组1 ==
  data: w_E input; dtau input; delta input; ddelta input; chi input; dchi input; gamma input; alpha input; dalpha input; beta input; dsigma output; p input; q input; r input
function dsigma = fcn(w_E,dtau,delta,ddelta,chi,dchi,gamma,alpha,dalpha,beta,p,q,r)

dsigma = -p*cos(alpha)*cos(beta) - q*sin(beta) - r*sin(alpha)*cos(beta) + dalpha*sin(beta)+ ...
        dchi*sin(gamma) - ddelta*sin(chi)*cos(gamma) + (dtau + w_E)*( cos(delta)*cos(chi)*cos(gamma) + sin(delta)*sin(gamma) );

== matlab function z8/Subsystem/角速率方程组1/角速率方程组 ==
  data: Ix input; Iy input; Iz input; l_AB input; dp output; m_AB input; dq output; dr output; n_AB input; p input; q input; r input
function [dp,dq,dr] = fcn(Ix,Iy,Iz,l_AB,m_AB,n_AB,p,q,r)

dp = ( Iy-Iz )*q*r/Ix + l_AB/Ix;
dq = ( Iz-Ix )*p*r/Iy + m_AB/Iy;
dr = ( Iz-Ix )*p*q/Iz + n_AB/Iz;

== matlab function z8/Subsystem/速度方程组1/速度方程组 ==
  data: D input; m input; g input; w_E input; L input; C input; R input; delta input; V input; chi input; dV output; gamma input; dchi output; dgamma output; sigma input
function [dV,dchi,dgamma] = fcn(D,m,g,w_E,L,C,R,delta,V,chi,gamma,sigma)

dV = -D/m - g*sin(gamma) + w_E^2*R*cos(delta)/( sin(gamma)*cos(delta) - cos(gamma)*sin(delta)*cos(chi) );
dchi = -( L*sin(sigma) - C*cos(sigma) )/( m*V*cos(gamma) ) + V*cos(gamma)*sin(chi)*tan(delta) / R + ...
        2*w_E*( sin(delta) - cos(delta)*tan(gamma)*cos(chi) ) +... 
        w_E^2*R*sin(delta)*cos(delta)*sin(chi) / ( V*cos(gamma) ); 
dgamma = ( L*cos(sigma) + C*sin(sigma) ) / ( m*V ) + ( V/R - g/V )*cos(gamma)+ ...
        2*w_E*cos(delta)*sin(chi) + ...
        w_E^2*R*cos(delta)*( cos(delta)*cos(gamma) + sin(delta)*sin(gamma)*cos(chi) )/V;

== matlab function z8/Subsystem/飞行器自身参数/飞行器本体参数1 ==
  data: S input; D output; rou input; C output; L output; C_D input; C_C input; C_L input; V input
function [D,C,L] = fcn(S,rou,C_D,C_C,C_L,V)

q_guji = 0.5*rou*V^2;

D = C_D*q_guji*S;    %阻力
C = C_C*q_guji*S;    %侧力
L = C_L*q_guji*S;    %升力

== matlab function z8/Subsystem/飞行器自身参数/飞行器本体参数2 ==
  data: m input; S input; c input; b input; l_AB output; rou input; C_l input; C_m input; C_n input; m_AB output; n_AB output; V input; alpha input; beta input; D input; C input; L input
function [l_AB,m_AB,n_AB] = fcn(m,S,c,b,rou,C_l,C_m,C_n,V,alpha,beta,D,C,L)

q_guji = 0.5*rou*V^2;

X_cg = 0.00000000016469*m^2 - 0.00005571500480*m + 7.36721170979675;

l_AB = C_l*q_guji*S*b;                                          %翻滚力矩
m_AB = C_m*q_guji*S*c + X_cg*( D*sin(alpha) + L*cos(alpha) );   %俯仰力矩
n_AB = C_n*q_guji*S*b + X_cg*C*cos(beta);                       %偏航力矩

== matlab function z8/Subsystem/飞行器自身参数/飞行器本体参数3 ==
  data: m input; Ix output; Iy output; Iz output
function [Ix,Iy,Iz] = fcn(m)

% Ix = -7.1*1e-5*m^2 + 19.91*m - 5.9340*1e4;
% Iy = -8.03*1e-4*m^2 + 219.74*m - 1.69*1e6;
% Iz = -8.03*1e-4*m^2 + 219.74*m - 1.69*1e6;

Ix = 1.0e+004*(-0.00000000709597*m^2 + 0.00199093623971*m - 5.94301903021396);
Iy = 1.0e+006*(-0.00000000080331*m^2 + 0.00021974209927*m - 1.69055469296301);
Iz = Iy;

== matlab function z8/MATLAB Function ==
  data: height input; aero_params output; velocity input; mach input; alpha_rad input; beta_rad input; le_deg input; re_deg input; rud_deg input; p_rads input; q_rads input; r_rads input; mass_kg input; atmosphere output
function [aero_params, atmosphere] = calculateAeroParameters(...
    height, velocity, mach, alpha_rad, beta_rad, ...
    le_deg, re_deg, rud_deg, p_rads, q_rads, r_rads, mass_kg)
% CALCULATEAEROPARAMETERS 计算飞行器气动参数和大气环境参数
%
% 输入参数:
%   height     - 几何高度 [m] (地心到飞行器质心距离减去地球半径)
%   velocity   - 飞行速度 [m/s]
%   mach       - 马赫数
%   alpha_rad  - 迎角 [rad]
%   beta_rad   - 侧滑角 [rad]
%   le_deg     - 左升降副翼偏角 [deg]
%   re_deg     - 右升降副翼偏角 [deg]
%   rud_deg    - 方向舵偏角 [deg]
%   p_rads     - 滚转角速率 [rad/s]
%   q_rads     - 俯仰角速率 [rad/s]
%   r_rads     - 偏航角速率 [rad/s]
%   mass_kg    - 飞行器质量 [kg]
%
% 输出参数:
%   aero_params - 结构体，包含所有气动系数和力/力矩
%   atmosphere  - 结构体，包含大气环境参数

    %% 初始化常数参数
    [d2r, S_ref, c_ref, b_ref, g, control_limits] = initConstants();
    
    %% 计算大气环境参数
    atmosphere = calculateAtmosphere(height);
    
    %% 计算动压
    q_bar = 0.5 * atmosphere.density * velocity^2;
    
    %% 计算气动系数
    aero_coeffs = calculateAeroCoefficients(...
        le_deg, re_deg, rud_deg, velocity, p_rads, q_rads, r_rads, ...
        mach, alpha_rad, beta_rad, d2r, c_ref, b_ref, control_limits);
    
    %% 计算气动力和力矩
    [forces, moments] = calculateForcesAndMoments(...
        aero_coeffs, q_bar, S_ref, c_ref, b_ref, alpha_rad, beta_rad, mass_kg);
    
    %% 组装输出结构体
    aero_params = struct();
    
    % 气动系数
    aero_params.CD = aero_coeffs.CD;
    aero_params.CL = aero_coeffs.CL;
    aero_params.CC = aero_coeffs.CY;  % 注意: CY就是侧力系数CC
    aero_params.Cl = aero_coeffs.Cll; % 滚转力矩系数
    aero_params.Cm = aero_coeffs.Cm;  % 俯仰力矩系数
    aero_params.Cn = aero_coeffs.Cn;  % 偏航力矩系数
    
    % 气动力 (N)
    aero_params.D = forces.D;  % 阻力
    aero_params.L = forces.L;  % 升力
    aero_params.C = forces.C;  % 侧力
    
    % 气动力矩 (N·m)
    aero_params.l = moments.l; % 滚转力矩
    aero_params.m = moments.m; % 俯仰力矩
    aero_params.n = moments.n; % 偏航力矩
    
    % 其他参数
    aero_params.q_bar = q_bar;        % 动压 [Pa]
    aero_params.LD = aero_coeffs.LD;  % 升阻比
    
    % 大气参数也放入aero_params便于访问
    aero_params.rho = atmosphere.density;
    aero_params.temperature = atmosphere.temperature;
    aero_params.pressure = atmosphere.pressure;
    aero_params.sound_speed = atmosphere.sound_speed;
end

%% 子函数: 初始化常数
function [d2r, S_ref, c_ref, b_ref, g, control_limits] = initConstants()
    d2r = pi/180;
    S_ref = 334.73;      % 参考机翼面积 [m²]
    c_ref = 24.384;      % 平均气动弦长 [m]
    b_ref = 18.288;      % 机翼展长 [m]
    g = 9.65;            % 重力加速度 [m/s²]
    
    % 操纵面偏转限制 [deg]
    control_limits.MAX_RE = 30;
    control_limits.MIN_RE = -30;
    control_limits.MAX_LE = 30;
    control_limits.MIN_LE = -30;
    control_limits.MAX_RUD = 30;
    control_limits.MIN_RUD = -30;
end

%% 子函数: 计算大气参数
function atmosphere = calculateAtmosphere(height)
    % 调用原始的大气模型函数
    air_quality = Sub_Height2AirQuality(height);
    
    atmosphere = struct();
    atmosphere.temperature = air_quality(1);    % [K]
    atmosphere.sound_speed = air_quality(2);    % [m/s]
    atmosphere.pressure = air_quality(3);       % [Pa]
    atmosphere.density = air_quality(4);        % [kg/m³]
end

%% 子函数: 计算气动系数
function coeffs = calculateAeroCoefficients(...
    LE, RE, RUD, V, p, q, r, MACH, alpha, beta, ...
    d2r, c_ref, b_ref, control_limits)

    % 角度转换
    ALP = alpha / d2r;  % 迎角转角度
    
    % 提取操纵面限制
    MAX_RE = control_limits.MAX_RE;
    MIN_RE = control_limits.MIN_RE;
    MAX_LE = control_limits.MAX_LE;
    MIN_LE = control_limits.MIN_LE;

    %% 阻力系数 CD
    CDa = 8.717E-02 - 3.307E-02*MACH + 3.179E-03*ALP - 1.250E-04*(ALP*MACH) + ...
          5.036E-03*MACH^2 - 1.100E-03*ALP^2 + 1.405E-07*(ALP*MACH)^2 - ...
          3.658E-04*MACH^3 + 3.175E-04*ALP^3 + 1.274E-05*MACH^4 - ...
          2.985E-05*ALP^4 - 1.705E-07*MACH^5 + 9.766E-07*ALP^5;
    
    CD_LE = 0;
    CD_RE = 0;
    CD_RUD = 0;
    
    coeffs.CD = CDa + CD_RE*RE + CD_LE*LE + CD_RUD*RUD;

    %% 升力系数 CL
    CLa = -8.19E-02 + 4.70E-02*MACH + 1.86E-02*ALP - 4.73E-04*(ALP*MACH) - ...
          9.19E-03*MACH^2 - 1.52E-04*ALP^2 + 5.99E-07*(ALP*MACH)^2 + ...
          7.74E-04*MACH^3 + 4.08E-06*ALP^3 - 2.93E-05*MACH^4 - ...
          3.91E-07*ALP^4 + 4.12E-07*MACH^5 + 1.30E-08*ALP^5;
    
    CL_LE = 0;
    CL_RE = 0;
    
    coeffs.CL = CLa + CL_RE*RE + CL_LE*LE;

    %% 俯仰力矩系数 Cm
    Cma = -2.192E-02 + 7.739E-03*MACH - 2.260E-03*ALP + 1.808E-04*(ALP*MACH) - ...
          8.849E-04*MACH^2 + 2.616E-04*ALP^2 - 2.880E-07*(ALP*MACH)^2 + ...
          4.617E-05*MACH^3 - 7.887E-05*ALP^3 - 1.143E-06*MACH^4 + ...
          8.288E-06*ALP^4 + 1.082E-08*MACH^5 - 2.789E-07*ALP^5;
    
    Cmq = -1.36E+00 + 3.86E-01*MACH + 7.85E-04*ALP + 1.40E-04*(ALP*MACH) - ...
          5.42E-02*MACH^2 + 2.36E-03*ALP^2 - 1.95E-06*(ALP*MACH)^2 + ...
          3.80E-03*MACH^3 - 1.48E-03*ALP^3 - 1.30E-04*MACH^4 + ...
          1.69E-04*ALP^4 + 1.71E-06*MACH^5 - 5.93E-06*ALP^5;
    
    Cm_LE = (0.0292/2)*d2r;
    Cm_RE = (0.0292/2)*d2r;
    Cm_RUD = 0;
    
    coeffs.Cm = Cma + Cm_RE*RE + Cm_LE*LE + Cm_RUD*RUD + Cmq*(q*c_ref)/(2*V);

    %% 侧力系数 CY (即CC)
    CYbv = -1.76E+00 + 4.58E-01*MACH - 3.26E-03*ALP + 3.80E-05*(ALP*MACH) - ...
           6.36E-02*MACH^2 + 2.36E-03*ALP^2 + 3.45E-07*(ALP*MACH)^2 + ...
           4.44E-03*MACH^3 - 6.03E-04*ALP^3 - 1.51E-04*MACH^4 + ...
           4.52E-05*ALP^4 + 1.98E-06*MACH^5 - 1.09E-06*ALP^5;
    
    % CY_RE 计算
    if RE <= 0
        temp = 2.27E-07*MIN_RE + 4.11E-09*(ALP*MACH)*MIN_RE - 5.04E-08*MIN_RE^2 + 4.50E-14*((ALP*MACH)*MIN_RE)^2;
        CY_RE = temp/MIN_RE;
    else
        temp = 2.27E-07*MAX_RE + 4.11E-09*(ALP*MACH)*MAX_RE - 5.04E-08*MAX_RE^2 + 4.50E-14*((ALP*MACH)*MAX_RE)^2;
        CY_RE = temp/MAX_RE;
    end
    
    % CY_LE 计算
    if LE <= 0
        temp = -(2.27E-07*MIN_LE + 4.11E-09*(ALP*MACH)*MIN_LE - 5.04E-08*MIN_LE^2 + 4.50E-14*((ALP*MACH)*MIN_LE)^2);
        CY_LE = temp/MIN_LE;
    else
        temp = -(2.27E-07*MAX_LE + 4.11E-09*(ALP*MACH)*MAX_LE - 5.04E-08*MAX_LE^2 + 4.50E-14*((ALP*MACH)*MAX_LE)^2);
        CY_LE = temp/MAX_LE;
    end
    
    CY_RUD = 3.84E-04 - 1.17E-05*ALP - 1.07E-05*MACH + 2.60E-07*(ALP*MACH);
    CYb = CYbv;
    
    coeffs.CY = CYb*beta + CY_RE*RE + CY_LE*LE + CY_RUD*RUD;

    %% 滚转力矩系数 Cl
    Cllbv = -1.402E-01 + 3.326E-02*MACH - 7.590E-04*ALP + 8.596E-06*(ALP*MACH) - ...
            3.794E-03*MACH^2 + 2.354E-06*ALP^2 - 1.044E-08*(ALP*MACH)^2 + ...
            2.219E-04*MACH^3 - 8.964E-18*ALP^3 - 6.462E-06*MACH^4 + ...
            3.803E-19*ALP^4 + 7.419E-08*MACH^5 - 3.353E-21*ALP^5;
    
    Cll_RE_AM = 3.570E-04 - 9.569E-05*ALP - 3.598E-05*MACH + 4.950E-06*ALP^2 + ...
                1.411E-06*MACH^2 - 3.4800e-004 - 1.3923e-008*(ALP*MACH)^2;
    Cll_RE = 1.170E-04 + 2.794E-08*(ALP*MACH);
    
    Cll_LE_AM = -(3.570E-04 - 9.569E-05*ALP - 3.598E-05*MACH + 4.950E-06*ALP^2 + ...
                  1.411E-06*MACH^2 - 3.4800e-004 - 1.3923e-008*(ALP*MACH)^2);
    Cll_LE = -(1.170E-04 + 2.794E-08*(ALP*MACH));
    
    Cll_RUD_AM = -5.0103E-19 + 6.2723E-20*ALP + 2.3418E-20*MACH - 3.4201E-21*(ALP*MACH);
    Cll_RUD = 0.00011441 - 2.6824E-06*ALP - 3.5496E-06*MACH + 5.5547E-08*(ALP*MACH);
    
    Cllr = 3.82E-01 - 1.06E-01*MACH + 1.94E-03*ALP - 8.15E-05*(ALP*MACH) + ...
           1.45E-02*MACH^2 - 9.76E-06*ALP^2 + 4.49E-08*(ALP*MACH)^2 - ...
           1.02E-03*MACH^3 - 2.70E-07*ALP^3 + 3.56E-05*MACH^4 + ...
           3.19E-08*ALP^4 - 4.81E-07*MACH^5 - 1.06E-09*ALP^5;
    
    Cllp = -2.99E-01 + 7.47E-02*MACH + 1.38E-03*ALP - 8.78E-05*(ALP*MACH) - ...
           9.13E-03*MACH^2 - 2.04E-04*ALP^2 - 1.52E-07*(ALP*MACH)^2 + ...
           5.73E-04*MACH^3 - 3.86E-05*ALP^3 - 1.79E-05*MACH^4 + ...
           4.21E-06*ALP^4 + 2.20E-07*MACH^5 - 1.15E-07*ALP^5;
    
    Cllb = Cllbv + Cll_RE_AM + Cll_LE_AM + Cll_RUD_AM;
    
    coeffs.Cll = Cllb*beta + Cll_RE*RE + Cll_LE*LE + Cll_RUD*RUD + ...
                 Cllr*(r*b_ref)/(2*V) + Cllp*(p*b_ref)/(2*V);

    %% 偏航力矩系数 Cn
    Cnbv = 3.68E-01 + 6.03E-16*ALP - 9.79E-02*MACH - 3.84E-16*ALP^2 + ...
           1.24E-02*MACH^2 + 8.58E-17*ALP^3 - 8.05E-04*MACH^3 - ...
           7.75E-18*ALP^4 + 2.57E-05*MACH^4 + 2.42E-19*ALP^5 - 3.20E-07*MACH^5;
    
    % Cn_RE 计算
    if RE <= 0
        Cn_RE_AM = 2.10E-04 + 1.83E-05*ALP - 3.56E-05*MACH - 6.39E-07*ALP^2 + 8.16E-07*MACH^2;
        temp = -1.30E-05*MIN_RE - 8.93E-08*(ALP*MACH)*MIN_RE + 1.97E-06*MIN_RE^2 + 1.41E-11*((ALP*MACH)*MIN_RE)^2;
        Cn_RE = temp/MIN_RE;
    else
        Cn_RE_AM = 2.10E-04 + 1.83E-05*ALP - 3.56E-05*MACH - 6.39E-07*ALP^2 + 8.16E-07*MACH^2;
        temp = -1.30E-05*MAX_RE - 8.93E-08*(ALP*MACH)*MAX_RE + 1.97E-06*MAX_RE^2 + 1.41E-11*((ALP*MACH)*MAX_RE)^2;
        Cn_RE = temp/MAX_RE;
    end
    
    % Cn_LE 计算
    if LE <= 0
        Cn_LE_AM = -(2.10E-04 + 1.83E-05*ALP - 3.56E-05*MACH - 6.39E-07*ALP^2 + 8.16E-07*MACH^2);
        temp = -(-1.30E-05*MIN_LE - 8.93E-08*(ALP*MACH)*MIN_LE + 1.97E-06*MIN_LE^2 + 1.41E-11*((ALP*MACH)*MIN_LE)^2);
        Cn_LE = temp/MIN_LE;
    else
        Cn_LE_AM = -(2.10E-04 + 1.83E-05*ALP - 3.56E-05*MACH - 6.39E-07*ALP^2 + 8.16E-07*MACH^2);
        temp = -(-1.30E-05*MAX_LE - 8.93E-08*(ALP*MACH)*MAX_LE + 1.97E-06*MAX_LE^2 + 1.41E-11*((ALP*MACH)*MAX_LE)^2);
        Cn_LE = temp/MAX_LE;
    end
    
    Cn_RUD_AM = 2.85E-18 - 3.59E-19*ALP - 1.26E-19*MACH + 1.57E-20*(ALP*MACH);
    Cn_RUD = -5.56E-03 + 2.78E-05*ALP + 3.30E-05*MACH - 6.26E-07*(ALP*MACH);
    
    Cnp = 3.68E-01 - 9.79E-02*MACH + 7.61E-16*ALP + 1.24E-02*MACH^2 - ...
          4.64E-16*ALP^2 - 8.05E-04*MACH^3 + 1.01E-16*ALP^3 + 2.57E-05*MACH^4 + ...
          -9.18E-18*ALP^4 - 3.20E-07*MACH^5 + 2.96E-19*ALP^5;
    
    Cnr = -2.41E+00 + 5.96E-01*MACH - 2.74E-03*ALP + 2.09E-04*(ALP*MACH) - ...
          7.57E-02*MACH^2 + 1.15E-03*ALP^2 - 6.53E-08*(ALP*MACH)^2 + ...
          4.90E-03*MACH^3 - 3.87E-04*ALP^3 - 1.57E-04*MACH^4 + ...
          3.60E-05*ALP^4 + 1.96E-06*MACH^5 - 1.18E-06*ALP^5;
    
    Cnb = Cnbv + Cn_RE_AM + Cn_LE_AM + Cn_RUD_AM;
    
    coeffs.Cn = Cnb*beta + Cn_RE*RE + Cn_LE*LE + Cn_RUD*RUD + ...
                Cnp*(p*b_ref)/(2*V) + Cnr*(r*b_ref)/(2*V);

    %% 升阻比
    coeffs.LD = coeffs.CL / coeffs.CD;
end

%% 子函数: 计算气动力和力矩
function [forces, moments] = calculateForcesAndMoments(...
    coeffs, q_bar, S_ref, c_ref, b_ref, alpha, beta, mass_kg)

    % 计算质心位置 (来自HSVmodel.m中的公式)
    X_cg = 1.65e-10 * mass_kg^2 - 5.57e-5 * mass_kg + 7.36721170979675;
    
    % 计算气动力
    forces.D = q_bar * S_ref * coeffs.CD;  % 阻力
    forces.C = q_bar * S_ref * coeffs.CY;  % 侧力
    forces.L = q_bar * S_ref * coeffs.CL;  % 升力
    
    % 计算气动力矩
    Z = forces.D * sin(alpha) + forces.L * cos(alpha);
    
    moments.l = q_bar * S_ref * b_ref * coeffs.Cll;                    % 滚转力矩
    moments.m = q_bar * S_ref * c_ref * coeffs.Cm + X_cg * Z;         % 俯仰力矩
    moments.n = q_bar * S_ref * b_ref * coeffs.Cn + X_cg * forces.C * cos(beta); % 偏航力矩
end

== matlab function z8/Subsystem/速度方程组12/速度方程组 ==
  data: D input; m input; g input; w_E input; L input; C input; R input; delta input; V input; chi input; dV output; gamma input; dchi output; dgamma output; sigma input
function [dV,dchi,dgamma] = fcn(D,m,g,w_E,L,C,R,delta,V,chi,gamma,sigma)

dV = -D/m - g*sin(gamma) + w_E^2*R*cos(delta)/( sin(gamma)*cos(delta) - cos(gamma)*sin(delta)*cos(chi) );
dchi = -( L*sin(sigma) - C*cos(sigma) )/( m*V*cos(gamma) ) + V*cos(gamma)*sin(chi)*tan(delta) / R + ...
        2*w_E*( sin(delta) - cos(delta)*tan(gamma)*cos(chi) ) +... 
        w_E^2*R*sin(delta)*cos(delta)*sin(chi) / ( V*cos(gamma) ); 
dgamma = ( L*cos(sigma) + C*sin(sigma) ) / ( m*V ) + ( V/R - g/V )*cos(gamma)+ ...
        2*w_E*cos(delta)*sin(chi) + ...
        w_E^2*R*cos(delta)*( cos(delta)*cos(gamma) + sin(delta)*sin(gamma)*cos(chi) )/V;

== matlab function z8/Subsystem/位置方程组12/位置方程组 ==
  data: R input; delta input; V input; chi input; dR output; gamma input; dtau output; ddelta output
function [dR,dtau,ddelta] = fcn(R,delta,V,chi,gamma)

dR = V*sin(gamma);
dtau = V*cos(gamma) * sin(chi) / ( R*cos(delta) );
ddelta = V*cos(gamma) * cos(chi) / R;

== matlab function z8/Subsystem/气流姿态角方程组12/气流姿态角方程组/气流姿态角方程组 ==
  data: w_E input; dtau input; delta input; ddelta input; chi input; dchi input; gamma input; dgamma input; alpha input; beta input; dalpha output; sigma input; dbeta output; p input; q input; r input
function [dalpha,dbeta] = fcn(w_E,dtau,delta,ddelta,chi,dchi,gamma,dgamma,alpha,beta,sigma,p,q,r)

dalpha = q - ( p*cos(alpha) + r*sin(alpha) )*tan(beta) + ...
        sin(sigma) / cos(beta) *( dchi*cos(gamma) - ddelta*sin(chi)*sin(gamma) + ( dtau + w_E )*( cos(delta)*cos(chi)*sin(gamma) - sin(delta)*cos(gamma) ) ) - ...
        cos(sigma) / cos(beta) *( dgamma - ddelta*cos(chi) - ( dtau + w_E )*cos(delta)*sin(chi) );
dbeta = p*sin(alpha) - r*cos(alpha) + sin(sigma)*( dgamma - ddelta*cos(chi) - ( dtau + w_E )*cos(delta)*sin(chi) ) + ...
        cos(sigma)*( dchi*cos(gamma) - ddelta*sin(chi)*sin(gamma) + ( dtau + w_E )*( cos(delta)*cos(chi)*sin(gamma) - sin(delta)*cos(gamma) ) );

== matlab function z8/Subsystem/气流姿态角方程组12/气流姿态角方程组/气流姿态角方程组1 ==
  data: w_E input; dtau input; delta input; ddelta input; chi input; dchi input; gamma input; alpha input; dalpha input; beta input; dsigma output; p input; q input; r input
function dsigma = fcn(w_E,dtau,delta,ddelta,chi,dchi,gamma,alpha,dalpha,beta,p,q,r)

dsigma = -p*cos(alpha)*cos(beta) - q*sin(beta) - r*sin(alpha)*cos(beta) + dalpha*sin(beta)+ ...
        dchi*sin(gamma) - ddelta*sin(chi)*cos(gamma) + (dtau + w_E)*( cos(delta)*cos(chi)*cos(gamma) + sin(delta)*sin(gamma) );
